simulink model "DynamicsOfManipulatorSim"  (Simulink 7.9)
settings: Solver=ode45  StartTime=0.0  StopTime=10  RelTol=1e-3
undefined symbols (not defined in the file or in its folder): u_max, u_min, x, xd, xdd
settings Model: Creator=Stepan  LastModifiedBy=katharina
settings DebuggingCC: FcnCallInpInsideContextMsg=Use local settings  StrictBusMsg=Warning
settings GRTTargetCC: CombineOutputUpdateFcns=off  GRTInterface=on

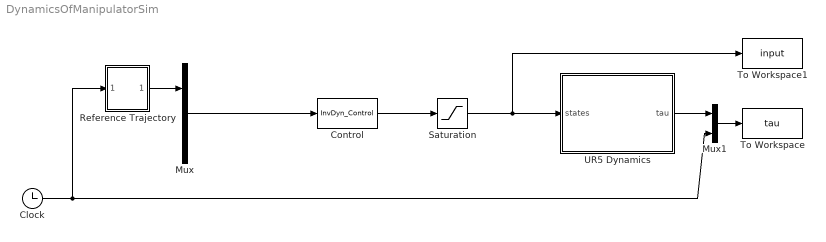
== system DynamicsOfManipulatorSim ==
  Clock : Clock
  Control : MATLABFcn  MATLABFcn=InvDyn_Control
  Mux : Mux  Inputs=[9;6;]
  Mux1 : Mux  Inputs=[6;1]
  Reference Trajectory : Subsystem
  Saturation : Saturate  UpperLimit=u_max  LowerLimit=u_min
  To Workspace : ToWorkspace  VariableName=tau  SampleTime=-1
  To Workspace1 : ToWorkspace  VariableName=input  SampleTime=-1
  UR5 Dynamics : Subsystem
  wires:
  Mux1/1 -> To Workspace/1
  Clock/1 -> Mux1/2, Reference Trajectory/1(In1)
  Control/1 -> Saturation/1
  Mux/1 -> Control/1
  Reference Trajectory/1(Out1) -> Mux/1
  Saturation/1 -> To Workspace1/1, UR5 Dynamics/1(states)
  UR5 Dynamics/1(tau) -> Mux1/1

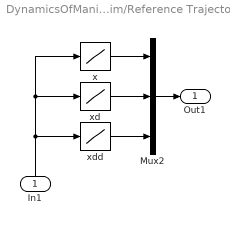
== system DynamicsOfManipulatorSim/Reference Trajectory ==
  In1 : Inport
  Mux2 : Mux  Inputs=3
  x : Lookup  InputValues=t  Table=x
  xd : Lookup  InputValues=t  Table=xd
  xdd : Lookup  InputValues=t  Table=xdd
  Out1 : Outport
  wires:
  x/1 -> Mux2/1
  xdd/1 -> Mux2/3
  In1/1 -> xdd/1, xd/1, x/1
  Mux2/1 -> Out1/1
  xd/1 -> Mux2/2

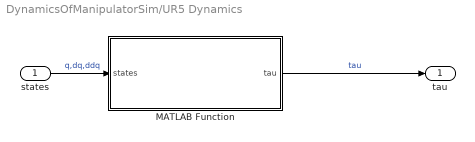
== system DynamicsOfManipulatorSim/UR5 Dynamics ==
  states : Inport
  MATLAB Function : MATLAB Function  TreatAsAtomicUnit=on
  tau : Outport
  wires:
  states/1 -> MATLAB Function/1(states)  "q,dq,ddq"
  MATLAB Function/1(tau) -> tau/1  "tau"

== matlab function UR5 Dynamics/MATLAB Function ==
  data: states input double; tau output double
function tau = ur5_ForwardDynamics(states)
%#codegen
q = states(1:6);
dq = states(7:12);
ddq = states(13:18);

[Mt, Gt, Ct_dq] = ur5_dynamics(q, dq);

tau = Mt*ddq + Ct_dq + Gt;

end
